simulink model "VehicleModel"  (R2016b)
settings: Solver=FixedStepAuto  StartTime=0.0  StopTime=t_EndSimulation  FixedStep=base_dT  MaxStep=0.01  RelTol=1e-3  EnableMultiTasking=on
values from neighbouring files (symbols this model uses):
  b_E2C_inloop = Simulink.Parameter    [VehicleModelInit.m]
  b_Engine_in_loop = Simulink.Parameter    [VehicleModelInit.m]
  b_initialize_distance_t_startsim = Simulink.Parameter    [VehicleModelInit.m]
  b_Ne_in_loop = Simulink.Parameter    [VehicleModelInit.m]
  b_TTB_in_loop = Simulink.Parameter    [VehicleModelInit.m]
  b_use_acc = Simulink.Parameter    [VehicleModelInit.m]
  b_use_acc_hardset = Simulink.Parameter    [VehicleModelInit.m]
  base_dT = Simulink.Parameter    [VehicleModelInit.m]
  c_acc_d_hdw = Simulink.Parameter    [VehicleModelInit.m]
  c_acc_hdw = Simulink.Parameter    [VehicleModelInit.m]
  c_EngFricCoef = PARS.c_EngFricCoef    [VehicleModelInit.m]
  c_EngFricCoefd = PARS.c_EngFricCoefd    [VehicleModelInit.m]
  d_Ne_max = Simulink.Parameter    [VehicleModelInit.m]
  d_Ne_min = Simulink.Parameter    [VehicleModelInit.m]
  Driver_TuneG1 = PARS.Driver_TuneG1    [VehicleModelInit.m]
  Driver_TuneG2 = PARS.Driver_TuneG2    [VehicleModelInit.m]
  Driver_TuneG3 = PARS.Driver_TuneG3    [VehicleModelInit.m]
  Driver_TuneG_aw = PARS.Driver_TuneG_aw    [VehicleModelInit.m]
  E2C_c2_dTB = Simulink.Parameter    [VehicleModelInit.m]
  E2C_c_dTB = Simulink.Parameter    [VehicleModelInit.m]
  E2C_CycleTimespan = Simulink.Parameter    [VehicleModelInit.m]
  E2C_initializeRelDist = Simulink.Parameter    [VehicleModelInit.m]
  E2C_SpeedShape = Simulink.Parameter    [VehicleModelInit.m]
  E2C_Trap_CycleAcceEndAlpha = Simulink.Parameter    [VehicleModelInit.m]
  E2C_Trap_CycleAcceStartAlpha = Simulink.Parameter    [VehicleModelInit.m]
  E2C_Trap_CycleDeceEndAlpha = Simulink.Parameter    [VehicleModelInit.m]
  E2C_Trap_CycleDeceStartAlpha = Simulink.Parameter    [VehicleModelInit.m]
  E2C_V_High_kmh = Simulink.Parameter    [VehicleModelInit.m]
  E2C_V_Low_kmh = Simulink.Parameter    [VehicleModelInit.m]
  E2C_V_max = Simulink.Parameter    [VehicleModelInit.m]
  E2C_V_min = Simulink.Parameter    [VehicleModelInit.m]
  FTP_speed_1sec = [FTP_speed_once.speed;Idle_speed_once;FTP_speed_once.speed;Idle_speed_once;FTP_speed_once.speed]    [VehicleModelInit.m]
  mass = 3123*1.3    (= 4059.9)    [VehicleModelInit.m]
  T_ACC_TuneG1_data = Simulink.Parameter    [VehicleModelInit.m]
  T_ACC_TuneG1_pt = Simulink.Parameter    [VehicleModelInit.m]
  T_ACC_TuneG2_data = Simulink.Parameter    [VehicleModelInit.m]
  T_ACC_TuneG2_pt = Simulink.Parameter    [VehicleModelInit.m]
  t_StartSimulation = Simulink.Parameter    [VehicleModelInit.m]
  T_TB_ego_ini = Simulink.Parameter    [VehicleModelInit.m]
  T_TB_OffSet = Simulink.Parameter    [VehicleModelInit.m]
  tau_EngTorque = Simulink.Parameter    [VehicleModelInit.m]
  tau_Ne = Simulink.Parameter    [VehicleModelInit.m]
  tau_pedal_dem = Simulink.Parameter    [VehicleModelInit.m]
  VESP_MD = x0.VESP    [VehicleModelInit.m]
undefined symbols (not defined in the file or in its folder): Continuous, DiscIntNeverNeededParam, initializeRelDist, p_ego_ini, p_lead_ini, PedalMapMD, r_w, Simulation_dT, spsSampleAndHoldModel, v_lead_ini, x0
libraries: simulink x9, spsEdgeDetectorModel x6, dspsigops x1
(part 2 of 7)

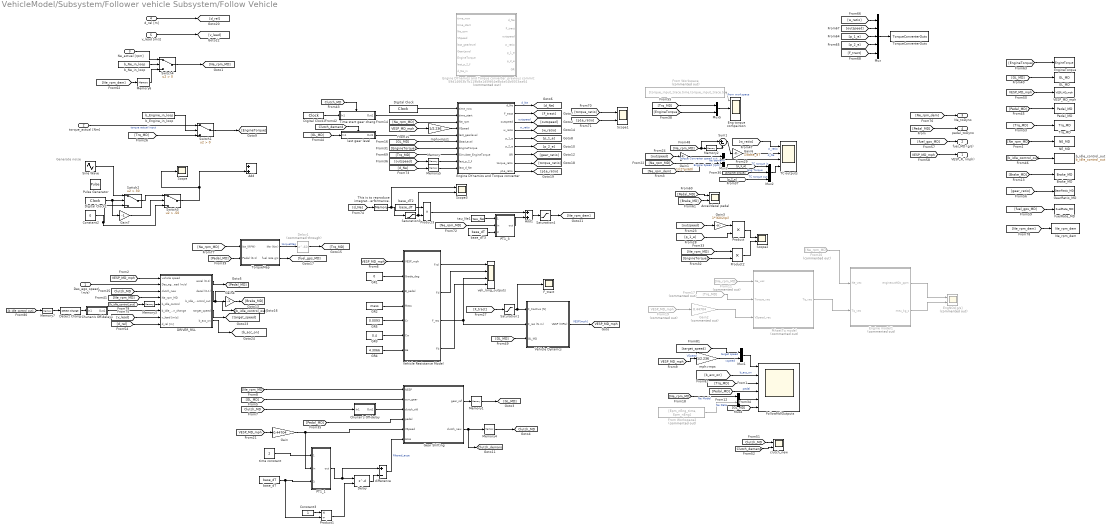
== system VehicleModel/Subsystem/Follower vehicle Subsystem/Follow Vehicle ==
  note: Generate noise
  Des_ego_speed (m/s) : Inport
  torque_actual [Nm] : Inport  Port=2
  Ne_actual [rpm] : Inport  Port=3
  d_rel [m] : Inport  Port=4
  v_lead [m/s] : Inport  Port=5
  Accel/decel pedal : Scope  NumInputPorts=2
  Add : Sum
  Add1 : Sum
  Brake_MD : ToWorkspace  VariableName=Brake_MD  SaveFormat=Structure With Time  SampleTime=-1
  Chunan's Off-delay : Subsystem
  Chunan's Off-delay1 : Subsystem
  Constant2 : Constant  Value=0
  Constant3 : Constant
  DRIVER_RSL : Subsystem
  Delay : Delay  DelayLengthSource=Input port  DelayLength=1
      settings: InputPortMap=u0,p1
  Delay1 : Delay  Commented=through  DelayLength=60
  Detect Change : simulink/Logic and Bit Operations/Detect Change  vinit=0  OutDataTypeStr=boolean
  Digital Clock : DigitalClock  SampleTime=-1
  Digital Clock1 : DigitalClock  SampleTime=-1
  Digital Clock2 : DigitalClock  SampleTime=-1
  Eng torque compairson : Scope  NumInputPorts=3
  EngNOx[g/s] : Scope  Commented=on  NumInputPorts=2
  Engine DYnamics and Torque converter : MATLAB Function  TreatAsAtomicUnit=on
  Engine DYnamics and Torque converter_previous commit: 59d14663b7b119b8a1d5fd64e8bda04b6003aa64 : MATLAB Function  Commented=on  TreatAsAtomicUnit=on
  Engine model1 : MATLAB Function  Commented=on  TreatAsAtomicUnit=on
  EngineTorque : ToWorkspace  VariableName=EngineTorque  SaveFormat=Structure With Time  SampleTime=-1
  F_tract : Scope
  FollowMdlOutputs : Scope  NumInputPorts=6
  From Workspace2 : FromWorkspace  Commented=on  VariableName=[Epm_nEng_time, Epm_nEng]
  From Workspace : FromWorkspace  Commented=on  VariableName=[torque_input_trace.time,torque_input_trace.tq]
  From11 : From  Commented=on  GotoTag=Ne_rpm_MD  TagVisibility=global
  From17 : From  Commented=on  GotoTag=Trq_MD  TagVisibility=global
  From19 : From  Commented=on  GotoTag=VESP_MD_mph  TagVisibility=global
  From20 : From  Commented=on  GotoTag=Ne_rpm_MD  TagVisibility=global
  FuelRate_MD : ToWorkspace  VariableName=FuelRate_MD  SaveFormat=Structure With Time  SampleTime=-1
  GL_MD : ToWorkspace  VariableName=GL_MD  SaveFormat=Structure With Time  SampleTime=-1
  GR1 : Constant  Value=0
  GR2 : Constant  Value=mass
  GR3 : Constant  Value=0.4
  GR4 : Constant  Value=4.3066
  GR5 : Constant  Value=0.0093
  Gain : Gain  Gain=0.44704
  Gain1 : Gain  Gain=1/(2*pi/60)
  Gain2 : Gain  Commented=on  Gain=0.44704
  Gain3 : Gain  Gain=1*(60/2/pi)
  Gain4 : Gain  Gain=-1
  Gain6 : Gain  Gain=1/base_dT
  Gain7 : Gain  Gain=-1
  Gear Shifting : MATLAB Function  TreatAsAtomicUnit=on
  GearRatio_MD : ToWorkspace  VariableName=GearRatio_MD  SaveFormat=Structure With Time  SampleTime=-1
  Memory{,3,5,7} (4 alike) : Memory  InheritSampleTime=on  LinearizeAsDelay=on
  Memory1 : Memory  X0=x0.GL  InheritSampleTime=on
  Memory2 : Memory  X0=600  InheritSampleTime=on  LinearizeAsDelay=on
  Memory4 : Memory  InheritSampleTime=on
  Memory6 : Memory  X0=600  InheritSampleTime=on  LinearizeAsDelay=on
  Mux : Mux  Inputs=5
  Mux1 : Mux  Inputs=2
  Mux2 : Mux  Inputs=3
  Mux3 : Mux  Inputs=3
  Mux4 : Mux  Inputs=2
  Mux5 : Mux  Inputs=2
  NE_MD : ToWorkspace  VariableName=NE_MD  SaveFormat=Structure With Time  SampleTime=-1
  Ne_rpm_dem : ToWorkspace  VariableName=Ne_rpm_dem  SaveFormat=Structure With Time  SampleTime=-1
  PT1_1 : Subsystem  mask(PT1_1){}
  PT1_3 : Subsystem  mask(PT1_1){}
  Pedal_MD : ToWorkspace  VariableName=Pedal_MD  SaveFormat=Structure With Time  SampleTime=-1
  Product : Product
  Product1 : Product  Inputs=*/
  Product2 : Product
  Product3 : Product
  PthsetTq model : MATLAB Function  Commented=on  TreatAsAtomicUnit=on
  Pulse Generator : DiscretePulseGenerator  Amplitude=250  Period=10  PulseWidth=5  SampleTime=-1
  Saturation1 : Saturate  UpperLimit=80000  LowerLimit=-80000
  Saturation3 : Saturate  UpperLimit=d_Ne_max  LowerLimit=d_Ne_min
  Saturation4 : Saturate  UpperLimit=3400  LowerLimit=600
  Scope : Scope
  Scope1 : Scope  NumInputPorts=2
  Scope2 : Scope  NumInputPorts=2
  Scope3 : Scope  NumInputPorts=2
  Sine Wave : Sin  Amplitude=0  Frequency=2
  Sum1 : Sum  Inputs=|+-
  Switch1 : Switch  Criteria=u2 > Threshold
  Switch2 : Switch  Criteria=u2 > Threshold  Threshold=30
  Switch3 : Switch  Criteria=u2 > Threshold  Threshold=-50
  Switch4 : Switch  Criteria=u2 > Threshold
  TC outputs : Scope  NumInputPorts=4
  This is to reproduce integrator performance. : Memory  InheritSampleTime=on  LinearizeAsDelay=on
  Time start gear change : Subsystem  TreatAsAtomicUnit=on
  TorqueConverterOuts : ToWorkspace  VariableName=TorqueConverterOuts  SaveFormat=Structure With Time  SampleTime=-1
  TorqueMap : Subsystem
  Trq_MD : ToWorkspace  VariableName=Trq_MD  SaveFormat=Structure With Time  SampleTime=-1
  VESP_MD_mph : ToWorkspace  VariableName=VESP_MD_mph  SaveFormat=Structure With Time  SampleTime=-1
  Vehicle Dynamcs : Subsystem
  Vehicle Resistance Model : MATLAB Function  TreatAsAtomicUnit=on
  b_Engine_in_loop : Constant  Value=b_Engine_in_loop
  b_Ne_in_loop : Constant  Value=b_Ne_in_loop
  b_idle_control_out : ToWorkspace  VariableName=b_idle_control_out  SaveFormat=Structure With Time  SampleTime=-1
  base_dT : Constant  Value=base_dT
  base_dT2 : Constant  Value=base_dT
  base_dT3 : Constant  Value=base_dT
  clutch_new : Scope  NumInputPorts=2
  difference : Sum  Inputs=+-  SaturateOnIntegerOverflow=on  InputSameDT=on  OutDataTypeStr=Inherit: Same as first input
  last gear level : Subsystem  TreatAsAtomicUnit=on
  mph>mps : Gain  Gain=1/2.236
  mph>mps1 : Gain  Gain=1/2.236
  tau_Ne1 : Constant  Value=tau_Ne
  time constant : Constant  Value=2
  veh_long_outputs : Scope  NumInputPorts=4
  VESP_FL (mph) : Outport
  fuel_MD (g/s) : Outport  Port=2
  Ne_toDyno : Outport  Port=3
  pedal_toDyno : Outport  Port=4
  tag scope: Clutch_MD=global, Clutch_demand=global, VESP_MD_mph=global
  wires:
  DRIVER_RSL/2(decel (0-1)) -> Gain4/1, Vehicle Resistance Model/3(B_pedal)
  Des_ego_speed (m/s)/1 -> DRIVER_RSL/2(Des_ego_speed (m/s))
  Vehicle Resistance Model/3(F_res) -> Vehicle Dynamcs/2(F_res (N.m)), veh_long_outputs/3
  GR1/1 -> Vehicle Resistance Model/2(Grade_deg)
  [VESP_MD_mph] -> Vehicle Resistance Model/1(VESP_mph)
  Vehicle Dynamcs/1(VESP (MPH)) -> [VESP_MD_mph]  "VESP[mph]"
  GR4/1 -> Vehicle Resistance Model/7(Aa)
  GR3/1 -> Vehicle Resistance Model/6(Cw)
  GR5/1 -> Vehicle Resistance Model/5(Cr)
  Vehicle Resistance Model/1(Frol) -> veh_long_outputs/1
  Vehicle Resistance Model/2(Fd) -> veh_long_outputs/2
  Vehicle Resistance Model/4(Fb) -> veh_long_outputs/4
  DRIVER_RSL/1(accel (0-1)) -> [Pedal_MD]
  [VESP_MD_mph] -> DRIVER_RSL/1(vehicle speed)
  [Ne_rpm_MD] -> TorqueMap/1(Ne_(RPM))
  TorqueMap/2(fuel rate g/s) -> [fuel_gps_MD]
  GR2/1 -> Vehicle Resistance Model/4(Mass)
  [GL_MD] -> Gear Shifting/2(curr_gear)
  [Ne_rpm_MD] -> Gear Shifting/1(NESP)
  Gear Shifting/1(gear_ref) -> Memory1/1
  Gear Shifting/2(clutch_new) -> Memory4/1, [Clutch_demand]
  [VESP_MD_mph] -> mph>mps/1  "VSpeed"
  [b_acc_on] -> FollowMdlOutputs/2  "b_acc_on"
  [Pedal_MD] -> FollowMdlOutputs/4  "pedal"
  Memory1/1 -> [GL_MD]
  [Trq_MD] -> FollowMdlOutputs/3
  Gain/1 -> PT1_1/2(in), Gear Shifting/5(VSpeed)
  [VESP_MD_mph] -> mph>mps1/1
  mph>mps1/1 -> Engine DYnamics and Torque converter/4(VSpeed)
  [GL_MD] -> Engine DYnamics and Torque converter/6(GearLevel)
  [EngineTorque] -> Mux2/2  "Eng Torque"
  Chunan's Off-delay/1(Out1) -> Gear Shifting/3(clutch_old)
  [Ne_rpm_MD] -> Engine DYnamics and Torque converter/3(Ne_rpm)
  [Ne_rpm_MD] -> Mux3/2  "Engine Speed [rpm]"
  Mux3/1 -> TC outputs/3
  From Workspace2/1 -> Mux4/2  "Ne Data"
  [Ne_rpm_MD] -> Mux4/1  "Ne Model"
  Mux4/1 -> FollowMdlOutputs/5
  From19/1 -> Gain2/1
  Gain2/1 -> PthsetTq model/3(VSpeed_vec)
  From17/1 -> PthsetTq model/2(Torque_vec)
  From11/1 -> PthsetTq model/1(Ne_vec)
  From20/1 -> Engine model1/1(Ne_vec)
  PthsetTq model/1(Tq_vec) -> Engine model1/2(Tq_vec)
  Engine model1/1(engineoutNOx_ppm) -> EngNOx[g/s]/1
  Engine model1/2(meu_kg_s) -> EngNOx[g/s]/2
  Engine DYnamics and Torque converter/1(d_Ne) -> [d_Ne]  "d_Ne"
  Engine DYnamics and Torque converter/3(outspeed) -> [outspeed]  "outspeed"
  [F_tract] -> Saturation1/1
  [VESP_MD_mph] -> Gain/1
  PT1_1/1(out) -> difference/1, Delay/1
  difference/1 -> Gear Shifting/6(Acce)  "filtered_acce"
  time constant/1 -> PT1_1/1(T_constant)
  Delay/1 -> difference/2
  Product1/1 -> Delay/2
  base_dT/1 -> Product1/2, PT1_1/3(T_sample)
  Constant3/1 -> Product1/1
  [Pedal_MD] -> pedal_toDyno/1
  Saturation1/1 -> F_tract/1, Vehicle Dynamcs/1(F_tractive [N])
  Product/1 -> Scope2/1
  Product2/1 -> Scope2/2
  Gain3/1 -> Product/1
  TorqueMap/1(Me (Nm)) -> Delay1/1  "torqueMap"
  b_Engine_in_loop/1 -> Switch1/2
  torque_actual [Nm]/1 -> Switch1/1  "torque actual input"
  [outspeed] -> Gain3/1
  [outspeed] -> Gain1/1
  Sum1/1 -> Gain6/1
  Engine DYnamics and Torque converter/2(F_tract) -> [F_tract]
  [p_1_e] -> Product/2
  [EngineTorque] -> Product2/2
  [Ne_rpm_MD] -> Product2/1
  [GL_MD] -> FollowMdlOutputs/6
  Gain4/1 -> [Brake_MD]
  [EngineTorque] -> Engine DYnamics and Torque converter/7(EngineTorque)
  Mux2/1 -> TC outputs/4
  [p_1_e] -> Mux2/1  "TC torque in"
  [p_2_e] -> Mux2/3  "TC torque out"
  Mux5/1 -> Eng torque compairson/2
  [Pedal_MD] -> TorqueMap/2(Pedal (0-1))
  [EngineTorque] -> Mux5/2
  From Workspace/1 -> Eng torque compairson/1  "from workspace"
  Gain1/1 -> Mux3/1  "Torque Converter speed out"
  [Ne_rpm_MD] -> Sum1/1, Memory2/1
  Memory2/1 -> Sum1/2
  [Clutch_MD] -> DRIVER_RSL/3(clutch_new)
  [Ne_rpm_MD] -> DRIVER_RSL/4(Ne_rpm_MD)
  Digital Clock/1 -> Engine DYnamics and Torque converter/1(time_now)
  [Clutch_MD] -> Chunan's Off-delay/1(In1)
  Memory4/1 -> [Clutch_MD]
  Digital Clock1/1 -> Time start gear change/1(In1)
  [Clutch_MD] -> Time start gear change/Trigger
  Time start gear change/1(Out1) -> Engine DYnamics and Torque converter/2(time_start)
  [Clutch_demand] -> last gear level/Trigger
  last gear level/1(Out1) -> Engine DYnamics and Torque converter/5(last_gearlevel)
  [GL_MD] -> last gear level/1(In1)
  [Trq_MD] -> Mux5/1
  Engine DYnamics and Torque converter/4(w_ratio) -> [w_ratio]  "w_ratio"
  [w_ratio] -> TC outputs/1  "w_ratio"
  Gain6/1 -> TC outputs/2  "d_Ne"
  [GL_MD] -> GL_MD/1
  [GL_MD] -> Vehicle Dynamcs/3(GL_MD)
  [VESP_MD_mph] -> VESP_MD_mph/1
  [Clutch_demand] -> clutch_new/2
  [Clutch_MD] -> clutch_new/1
  [Trq_MD] -> Trq_MD/1
  [Pedal_MD] -> Pedal_MD/1
  [Ne_rpm_MD] -> NE_MD/1
  [Brake_MD] -> Brake_MD/1
  [Pedal_MD] -> Gear Shifting/4(pedal)
  DRIVER_RSL/3(b_idle_control_out) -> [b_idle_control_out]
  [b_idle_control_out] -> b_idle_control_out/1
  [gear_ratio] -> GearRatio_MD/1
  [fuel_gps_MD] -> fuel_MD (g/s)/1
  [VESP_MD_mph] -> VESP_FL (mph)/1
  [fuel_gps_MD] -> FuelRate_MD/1
  [Brake_MD] -> Accel/decel pedal/2
  [Pedal_MD] -> Accel/decel pedal/1
  [Ne_rpm_dem] -> Ne_toDyno/1
  [Trq_MD] -> Switch1/3
  [EngineTorque] -> EngineTorque/1
  Mux/1 -> TorqueConverterOuts/1
  [w_ratio] -> Mux/1
  [outspeed] -> Mux/2
  [p_1_e] -> Mux/3
  [p_2_e] -> Mux/4
  [F_tract] -> Mux/5
  Digital Clock2/1 -> Gain7/1, Switch2/2
  Gain7/1 -> Switch3/2
  Sine Wave/1 -> Switch2/1
  Switch2/1 -> Switch3/1
  Constant2/1 -> Switch3/3, Switch2/3
  Switch3/1 -> Scope/1, Add/2
  Engine DYnamics and Torque converter/7(GR) -> [gear_ratio]
  Engine DYnamics and Torque converter/6(p_2_e) -> [p_2_e]
  Engine DYnamics and Torque converter/5(p_1_e) -> [p_1_e]
  Engine DYnamics and Torque converter/8(torque_ratio) -> [torque_ratio]
  Engine DYnamics and Torque converter/9(p1e_ratio) -> [p1e_ratio]
  [torque_ratio] -> Scope1/1
  [p1e_ratio] -> Scope1/2
  [outspeed] -> Memory/1
  Memory/1 -> Engine DYnamics and Torque converter/9(last_p_2_f)
  [d_Ne] -> Memory5/1
  Memory5/1 -> Engine DYnamics and Torque converter/10(last_d_Ne)
  [Trq_MD] -> Engine DYnamics and Torque converter/8(Simulate_EngineTorque)
  Switch1/1 -> [EngineTorque]
  [d_Ne] -> This is to reproduce integrator performance./1
  Product3/1 -> Add1/1
  Saturation3/1 -> Scope3/2, Product3/2
  base_dT2/1 -> Product3/1
  Add1/1 -> Saturation4/1
  Saturation4/1 -> [Ne_rpm_dem]
  [Ne_rpm_dem] -> Memory6/1
  This is to reproduce integrator performance./1 -> Scope3/1, Saturation3/1
  [Ne_rpm_dem] -> Mux3/3  "Ne demand"
  b_Ne_in_loop/1 -> Switch4/2
  Ne_actual [rpm]/1 -> Switch4/1
  Switch4/1 -> [Ne_rpm_MD]
  Memory6/1 -> Switch4/3
  [Ne_rpm_dem] -> Ne_rpm_dem/1
  tau_Ne1/1 -> PT1_3/1(T_constant)
  base_dT3/1 -> PT1_3/3(T_sample)
  [Ne_rpm_MD] -> PT1_3/2(in)
  PT1_3/1(out) -> Add1/2
  d_rel [m]/1 -> [d_rel]
  v_lead [m/s]/1 -> [v_lead]
  [d_rel] -> DRIVER_RSL/8(d_rel [m])
  [v_lead] -> DRIVER_RSL/7(v_lead [m/s])
  Chunan's Off-delay1/1(Out1) -> DRIVER_RSL/6(b_idle_is_in_change)
  Detect Change/1 -> Chunan's Off-delay1/1(In1)
  Delay1/1 -> [Trq_MD]
  [b_idle_control_out] -> Memory3/1
  Memory3/1 -> DRIVER_RSL/5(b_idle_control)
  [b_idle_control_out] -> Memory7/1
  Memory7/1 -> Detect Change/1
  DRIVER_RSL/4(target_speed) -> [target_speed]
  [target_speed] -> Mux1/1  "target speed"
  Mux1/1 -> FollowMdlOutputs/1
  mph>mps/1 -> Mux1/2  "vspeed"
  DRIVER_RSL/5("b_acc_on ") -> [b_acc_on]

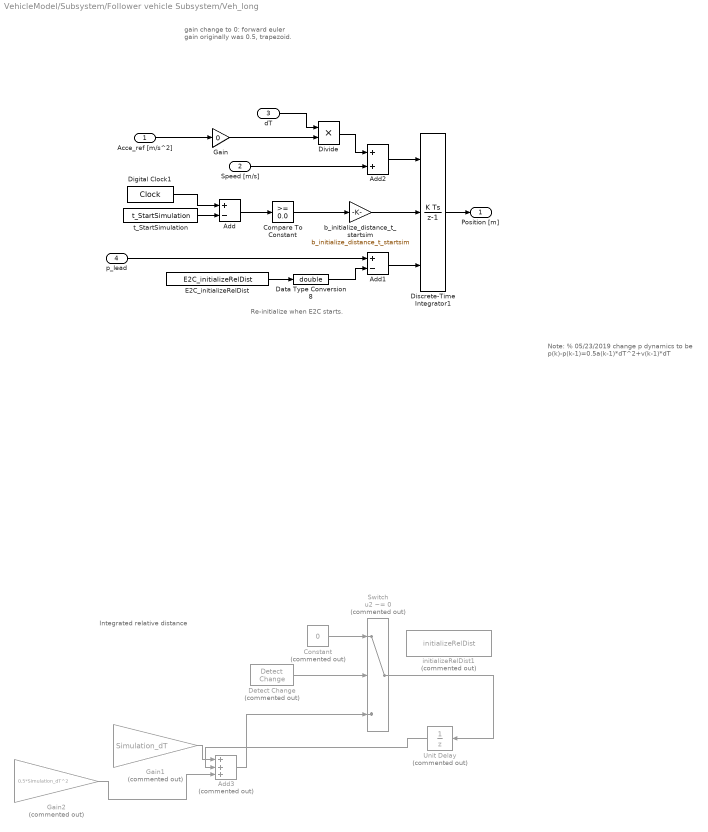
== system VehicleModel/Subsystem/Follower vehicle Subsystem/Veh_long  ==
  note: Re-initialize when E2C starts.
  note: gain change to 0: forward euler
      | gain originally was 0.5, trapezoid.
  note: Note:
      | % 05/23/2019
      | change p dynamics to be p(k)-p(k-1)=0.5a(k-1)*dT^2+v(k-1)*dT
  note: Integrated relative distance
  Acce_ref [m/s^2] : Inport
  Speed [m/s] : Inport  Port=2
  dT : Inport  Port=3
  p_lead : Inport  Port=4
  Add : Sum  Inputs=+-
  Add1 : Sum  Inputs=+-
  Add2 : Sum
  Add3 : Sum  Commented=on  Inputs=+++
  Compare To Constant : simulink/Logic and Bit Operations/Compare To Constant  relop=>=  const=0.0  OutDataTypeStr=uint8
  Constant : Constant  Commented=on  Value=0
  Data Type Conversion8 : DataTypeConversion  OutDataTypeStr=double
  Detect Change : simulink/Logic and Bit Operations/Detect Change  Commented=on  vinit=0  OutDataTypeStr=boolean
  Digital Clock1 : DigitalClock  SampleTime=-1
  Discrete-Time Integrator1 : DiscreteIntegrator  ExternalReset=rising  InitialConditionSource=external  InitialCondition=p_ego_ini  SampleTime=-1  ICPrevOutput=DiscIntNeverNeededParam  ICPrevScaledInput=DiscIntNeverNeededParam
  Divide : Product  Inputs=**
  E2C_initializeRelDist : Constant  Value=E2C_initializeRelDist  OutDataTypeStr=double
  Gain : Gain  Gain=0
  Gain1 : Gain  Commented=on  Gain=Simulation_dT
  Gain2 : Gain  Commented=on  Gain=0.5*Simulation_dT^2
  Switch : Switch  Commented=on  Criteria=u2 ~= 0
  Unit Delay : UnitDelay  Commented=on  SampleTime=-1
  b_initialize_distance_t_startsim : Gain  Gain=b_initialize_distance_t_startsim
  initializeRelDist1 : Constant  Commented=on  Value=initializeRelDist
  t_StartSimulation : Constant  Value=t_StartSimulation
  Position [m] : Outport
  wires:
  Divide/1 -> Add2/1
  Add2/1 -> Discrete-Time Integrator1/1
  Switch/1 -> Unit Delay/1
  Detect Change/1 -> Switch/2
  Add3/1 -> Switch/3
  Unit Delay/1 -> Add3/2
  Gain1/1 -> Add3/1
  Constant/1 -> Switch/1
  Gain2/1 -> Add3/3
  Discrete-Time Integrator1/1 -> Position [m]/1
  Add1/1 -> Discrete-Time Integrator1/3
  Speed [m/s]/1 -> Add2/2
  Acce_ref [m/s^2]/1 -> Gain/1
  E2C_initializeRelDist/1 -> Data Type Conversion8/1
  Gain/1 -> Divide/2
  dT/1 -> Divide/1
  Add/1 -> Compare To Constant/1
  t_StartSimulation/1 -> Add/2
  Digital Clock1/1 -> Add/1
  Compare To Constant/1 -> b_initialize_distance_t_startsim/1
  p_lead/1 -> Add1/1
  Data Type Conversion8/1 -> Add1/2
  b_initialize_distance_t_startsim/1 -> Discrete-Time Integrator1/2

== system VehicleModel/Subsystem/Lead_Veh_long/noequal ==
  In1 : Inport
  Relational Operator : RelationalOperator  Operator=~=  OutDataTypeStr=boolean  RndMeth=Simplest
  Unit Delay : UnitDelay  SampleTime=-1
  Out1 : Outport
  wires:
  Relational Operator/1 -> Out1/1
  Unit Delay/1 -> Relational Operator/2
  In1/1 -> Unit Delay/1, Relational Operator/1

== system VehicleModel/Subsystem/Follower vehicle Subsystem/Follow Vehicle/Chunan's Off-delay ==
  In1 : Inport
  Constant : Constant
  Constant2 : Constant  Value=0
  Data Type Conversion1 : DataTypeConversion  OutDataTypeStr=boolean  SaturateOnIntegerOverflow=on  RndMeth=Zero
  Digital Clock : DigitalClock  SampleTime=-1
  Logical Operator4 : Logic  Operator=NOT  Inputs=1
  OFF Delay : Subsystem  AncestorBlock=spsOnOffDelayModel/Continuous/OFF Delay  TreatAsAtomicUnit=on
  Relational Operator1 : RelationalOperator  Operator===  RndMeth=Nearest  InputSameDT=on
  delay length : Constant  Value=2
  Out1 : Outport
  wires:
  OFF Delay/1(OUT) -> Out1/1
  Logical Operator4/1 -> OFF Delay/Enable
  Constant2/1 -> Relational Operator1/1
  Relational Operator1/1 -> Logical Operator4/1
  Constant/1 -> Relational Operator1/2
  Data Type Conversion1/1 -> OFF Delay/1(IN)
  Digital Clock/1 -> OFF Delay/2(clock)
  delay length/1 -> OFF Delay/3(DELAY)
  In1/1 -> Data Type Conversion1/1

== system VehicleModel/Subsystem/Follower vehicle Subsystem/Follow Vehicle/Chunan's Off-delay1 ==
  In1 : Inport
  Constant : Constant
  Constant2 : Constant  Value=0
  Data Type Conversion1 : DataTypeConversion  OutDataTypeStr=boolean  SaturateOnIntegerOverflow=on  RndMeth=Zero
  Digital Clock : DigitalClock  SampleTime=-1
  Logical Operator4 : Logic  Operator=NOT  Inputs=1
  OFF Delay : Subsystem  AncestorBlock=spsOnOffDelayModel/Continuous/OFF Delay  TreatAsAtomicUnit=on
  Relational Operator1 : RelationalOperator  Operator===  RndMeth=Nearest  InputSameDT=on
  delay length : Constant
  Out1 : Outport
  wires:
  OFF Delay/1(OUT) -> Out1/1
  Logical Operator4/1 -> OFF Delay/Enable
  Constant2/1 -> Relational Operator1/1
  Relational Operator1/1 -> Logical Operator4/1
  Constant/1 -> Relational Operator1/2
  Data Type Conversion1/1 -> OFF Delay/1(IN)
  Digital Clock/1 -> OFF Delay/2(clock)
  delay length/1 -> OFF Delay/3(DELAY)
  In1/1 -> Data Type Conversion1/1

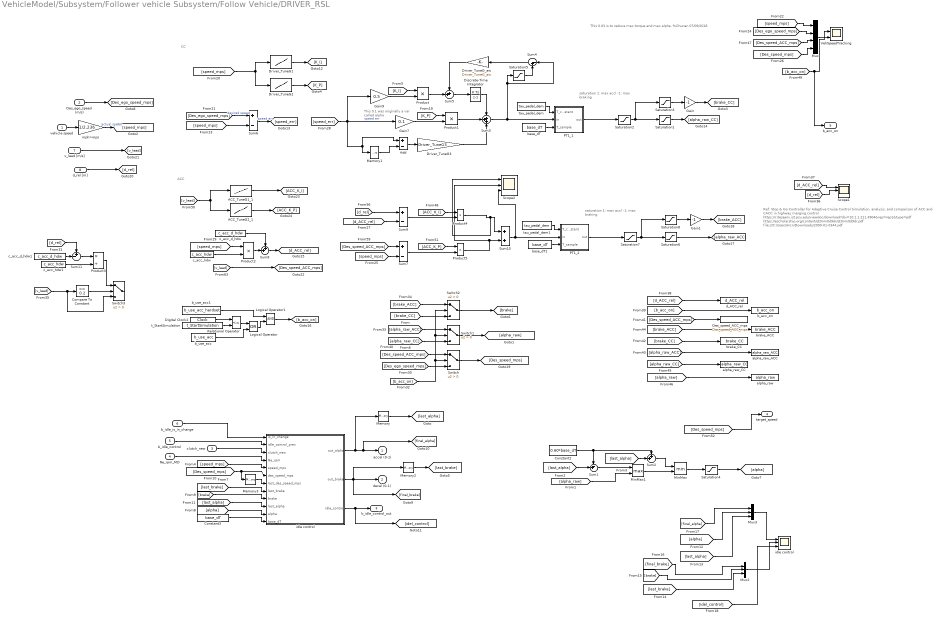
== system VehicleModel/Subsystem/Follower vehicle Subsystem/Follow Vehicle/DRIVER_RSL ==
  note: ACC
  note: CC
  note: Ref:
      | Stop & Go Controller for Adaptive Cruise Control
      | Simulation, analysis, and comparison of ACC and CACC in highway merging control
      | https://citeseerx.ist.psu.edu/viewdoc/download?doi=10.1.1.211.4904&rep=rep1&type=pdf
      | https://escholarship.org/content/qt0nm0d9dr/qt0nm0d9dr.pdf
      | file:///C:/Users/Hcn/Downloads/2000-01-0344.pdf
  note: This 0.1 was originally a var called alpha
  note: saturation
      | 1: max accl
      | -1: max braking
  note: This 0.03 is to reduce max torque and max alpha. %Chunan 07/09/2018
  note: saturation
      | 1: max accl
      | -1: max braking
  vehicle speed : Inport
  Des_ego_speed (m/s) : Inport  Port=2
  clutch_new : Inport  Port=3
  Ne_rpm_MD : Inport  Port=4
  b_idle_control : Inport  Port=5
  b_idle_is_in_change : Inport  Port=6
  v_lead [m/s] : Inport  Port=7
  d_rel [m] : Inport  Port=8
  ACC_TuneG1_1 : Lookup_n-D  NumberOfTableDimensions=1  BreakpointsForDimension1=T_ACC_TuneG1_pt  Table=T_ACC_TuneG1_data  InternalRulePriority=Speed  RndMeth=Simplest  InputSameDT=on
  ACC_TuneG2_1 : Lookup_n-D  NumberOfTableDimensions=1  BreakpointsForDimension1=T_ACC_TuneG2_pt  Table=T_ACC_TuneG2_data  InternalRulePriority=Speed  RndMeth=Simplest  InputSameDT=on
  Add : Sum  Inputs=+-
  Compare To Constant : simulink/Logic and Bit Operations/Compare To Constant  relop=>=  const=0.2  OutDataTypeStr=boolean
  Constant2 : Constant  Value=0.60*base_dT
  Constant3 : Constant  Value=base_dT
  Des_speed_ACC_mps : ToWorkspace  VariableName=Des_speed_ACC_mps  SaveFormat=Structure With Time  SampleTime=-1
  Digital Clock2 : DigitalClock  SampleTime=-1
  Discrete-Time Integrator : DiscreteIntegrator  gainval=1  InitialConditionSetting=State (most efficient)  SampleTime=-1  ICPrevOutput=DiscIntNeverNeededParam  ICPrevScaledInput=DiscIntNeverNeededParam
  Driver_TuneG1 : Lookup_n-D  NumberOfTableDimensions=1  BreakpointsForDimension1=[-1, 0.5, 3, 8.1, 50]  Table=[Driver_TuneG1*3,Driver_TuneG1*2.5, Driver_TuneG1*2, Driver_TuneG1, Driver_TuneG1]  InternalRulePriority=Speed  RndMeth=Simplest  InputSameDT=on
  Driver_TuneG2 : Lookup_n-D  NumberOfTableDimensions=1  BreakpointsForDimension1=[-1,0.5, 3, 8.1, 50]  Table=[Driver_TuneG2*6, Driver_TuneG2*3, Driver_TuneG2*2, Driver_TuneG2, Driver_TuneG2]  InternalRulePriority=Speed  RndMeth=Simplest  InputSameDT=on
  Driver_TuneG3 : Gain  Gain=Driver_TuneG3  SaturateOnIntegerOverflow=on  OutDataTypeStr=Inherit: Same as input  ParamDataTypeStr=Inherit: Same as input
  Driver_TuneG_aw : Gain  Gain=Driver_TuneG_aw
  Gain : Gain  Gain=-1  SaturateOnIntegerOverflow=on  OutDataTypeStr=Inherit: Same as input  ParamDataTypeStr=Inherit: Same as input
  Gain1 : Gain  Gain=-1  SaturateOnIntegerOverflow=on  OutDataTypeStr=Inherit: Same as input  ParamDataTypeStr=Inherit: Same as input
  Gain7 : Gain  Gain=0.1  SaturateOnIntegerOverflow=on  OutDataTypeStr=Inherit: Same as input  ParamDataTypeStr=Inherit: Same as input
  Gain9 : Gain  Gain=0.5  SaturateOnIntegerOverflow=on  OutDataTypeStr=Inherit: Same as input  ParamDataTypeStr=Inherit: Same as input
  Logical Operator : Logic  Operator=OR  AllPortsSameDT=off  OutDataTypeStr=boolean
  Logical Operator1 : Logic  AllPortsSameDT=off  OutDataTypeStr=boolean
  Memory{,1..3} (4 alike) : Memory  InheritSampleTime=on  LinearizeAsDelay=on
  MinMax : MinMax  Inputs=2
  MinMax1 : MinMax  Function=max  Inputs=2
  Mux : Mux
  Mux2 : Mux  Inputs=3
  Mux3 : Mux  Inputs=3
  PT1_1 : Subsystem  mask(PT1_1){}
  PT1_2 : Subsystem  mask(PT1_1){}
  Product{,1,4..5} (4 alike) : Product
  Product2 : Product  Inputs=**
  Product3 : Product  Inputs=*/
  Relational Operator : RelationalOperator  Operator=<=  OutDataTypeStr=boolean  RndMeth=Simplest
  Saturation1 : Saturate  UpperLimit=1  LowerLimit=0
  Saturation2 : Saturate  UpperLimit=1  LowerLimit=-1
  Saturation3 : Saturate  UpperLimit=0  LowerLimit=-1
  Saturation4 : Saturate  UpperLimit=1  LowerLimit=0
  Saturation5 : Saturate  UpperLimit=1  LowerLimit=-1
  Saturation6 : Saturate  UpperLimit=1  LowerLimit=0
  Saturation7 : Saturate  UpperLimit=1  LowerLimit=-1
  Saturation8 : Saturate  UpperLimit=0  LowerLimit=-1
  Scope1 : Scope  NumInputPorts=3
  Scope2 : Scope  NumInputPorts=3
  Sum1 : Sum  Inputs=-+|
  Sum10 : Sum  SaturateOnIntegerOverflow=on  InputSameDT=on  OutDataTypeStr=Inherit: Same as first input
  Sum11 : Sum  Inputs=+-|
  Sum2 : Sum  Inputs=++|
  Sum3 : Sum  Inputs=+++
  Sum4 : Sum  Inputs=|-+
  Sum5 : Sum  Inputs=++|
  Sum6 : Sum  Inputs=+-  SaturateOnIntegerOverflow=on  InputSameDT=on  OutDataTypeStr=Inherit: Same as first input
  Sum7 : Sum  Inputs=+-  SaturateOnIntegerOverflow=on  InputSameDT=on  OutDataTypeStr=Inherit: Same as first input
  Sum8 : Sum  Inputs=++|
  Sum9 : Sum  Inputs=+-  SaturateOnIntegerOverflow=on  InputSameDT=on  OutDataTypeStr=Inherit: Same as first input
  Switch{,1..3} (4 alike) : Switch  Criteria=u2 > Threshold
  VehSpeedTracking : Scope  NumInputPorts=2
  alpha_raw : ToWorkspace  VariableName=alpha_raw  SaveFormat=Structure With Time  SampleTime=-1
  alpha_raw_ACC : ToWorkspace  VariableName=alpha_raw_ACC  SaveFormat=Structure With Time  SampleTime=-1
  alpha_raw_CC : ToWorkspace  VariableName=alpha_raw_CC  SaveFormat=Structure With Time  SampleTime=-1
  b_acc_on : ToWorkspace  VariableName=b_acc_on  SaveFormat=Structure With Time  SampleTime=-1
  b_use_acc : Constant  Value=b_use_acc
  b_use_acc1 : Constant  Value=b_use_acc_hardset
  base_dT : Constant  Value=base_dT
  base_dT1 : Constant  Value=base_dT
  brake_ACC : ToWorkspace  VariableName=brake_ACC  SaveFormat=Structure With Time  SampleTime=-1
  brake_CC : ToWorkspace  VariableName=brake_CC  SaveFormat=Structure With Time  SampleTime=-1
  c_acc_d_hdw : Constant  Value=c_acc_d_hdw
  c_acc_d_hdw1 : Constant  Value=c_acc_d_hdw
  c_acc_hdw : Constant  Value=c_acc_hdw
  c_acc_hdw1 : Constant  Value=c_acc_hdw
  d_ACC_rel : ToWorkspace  VariableName=d_ACC_rel  SaveFormat=Structure With Time  SampleTime=-1
  idle control : MATLAB Function  TreatAsAtomicUnit=on
  "idle control " : Scope  NumInputPorts=3
  mph>mps : Gain  Gain=1/2.236
  t_StartSimulation : Constant  Value=t_StartSimulation
  tau_pedal_dem : Constant  Value=tau_pedal_dem
  tau_pedal_dem1 : Constant  Value=tau_pedal_dem
  accel (0-1) : Outport
  decel (0-1) : Outport  Port=2
  b_idle_control_out : Outport  Port=3
  target_speed : Outport  Port=4
  "b_acc_on " : Outport  Port=5
  wires:
  Gain/1 -> [brake_CC]
  Saturation3/1 -> Gain/1
  Saturation1/1 -> [alpha_raw_CC]
  vehicle speed/1 -> mph>mps/1
  Mux/1 -> VehSpeedTracking/1
  Saturation2/1 -> Saturation3/1, Saturation1/1
  Gain7/1 -> Product1/2
  Gain9/1 -> Product/2
  [Des_ego_speed_mps] -> Sum6/1  "desired speed"
  mph>mps/1 -> [speed_mps]  "actual speed"
  [speed_err] -> Gain7/1, Add/1, Memory1/1, Gain9/1  "speed err"
  Product/1 -> Sum5/2
  tau_pedal_dem/1 -> PT1_1/1(T_constant)
  base_dT/1 -> PT1_1/3(T_sample)
  PT1_1/1(out) -> Saturation2/1
  Memory/1 -> [last_alpha]
  MinMax/1 -> Saturation4/1
  [alpha_raw] -> MinMax1/2
  Saturation4/1 -> [alpha]
  [last_alpha] -> Sum1/2
  Constant2/1 -> Sum1/1, Sum2/1
  Sum1/1 -> MinMax1/1
  [last_alpha] -> Sum2/2
  MinMax1/1 -> MinMax/2
  Sum2/1 -> MinMax/1
  Memory1/1 -> Add/2
  Add/1 -> Driver_TuneG3/1
  Driver_TuneG3/1 -> Sum3/3
  Product1/1 -> Sum3/2
  Discrete-Time Integrator/1 -> Sum3/1
  Sum3/1 -> Sum4/1, Saturation5/1, PT1_1/2(in)
  Saturation5/1 -> Sum4/2
  Sum4/1 -> Driver_TuneG_aw/1
  Driver_TuneG_aw/1 -> Sum5/1
  Sum5/1 -> Discrete-Time Integrator/1
  Memory2/1 -> [last_brake]
  [alpha] -> idle control/11(alpha)
  [last_brake] -> idle control/8(last_brake)
  [speed_mps] -> idle control/5(speed_mps)
  Ne_rpm_MD/1 -> idle control/4(Ne_rpm)
  clutch_new/1 -> idle control/3(clutch_new)
  b_idle_control/1 -> idle control/2(idle_control_prev)
  [brake] -> idle control/9(brake)
  [Des_speed_mps] -> Memory3/1, idle control/6(des_speed_mps)
  [last_alpha] -> idle control/10(last_alpha)
  Constant3/1 -> idle control/12(base_dT)
  idle control/1(out_alpha) -> Memory/1, [final_alpha], accel (0-1)/1
  idle control/2(out_brake) -> [final_brake], Memory2/1, decel (0-1)/1
  idle control/3(idle_control) -> [idel_control], b_idle_control_out/1
  Mux2/1 -> "idle control "/2
  [final_brake] -> Mux2/1
  [brake] -> Mux2/2
  [last_brake] -> Mux2/3
  Mux3/1 -> "idle control "/1
  [last_alpha] -> Mux3/3
  [alpha] -> Mux3/2
  [final_alpha] -> Mux3/1
  [idel_control] -> "idle control "/3
  Memory3/1 -> idle control/7(last_des_speed_mps)
  Driver_TuneG1/1 -> [K_I]
  [K_I] -> Product/1
  Driver_TuneG2/1 -> [K_P]
  [K_P] -> Product1/1
  [speed_mps] -> Driver_TuneG2/1, Driver_TuneG1/1
  Des_ego_speed (m/s)/1 -> [Des_ego_speed_mps]
  [speed_mps] -> Mux/1
  [speed_mps] -> Sum6/2
  [Des_ego_speed_mps] -> Mux/2
  Sum6/1 -> [speed_err]  "speed err"
  Switch2/1 -> [brake]
  Switch1/1 -> [alpha_raw]
  [speed_mps] -> Sum7/2
  c_acc_hdw/1 -> Product2/2
  Sum8/1 -> [d_ACC_rel]
  c_acc_d_hdw/1 -> Sum8/1
  [speed_mps] -> Product2/1
  Product2/1 -> Sum8/2
  t_StartSimulation/1 -> Relational Operator/2
  Digital Clock2/1 -> Relational Operator/1
  Relational Operator/1 -> Logical Operator/1
  b_use_acc/1 -> Logical Operator/2
  Logical Operator/1 -> Logical Operator1/2
  b_use_acc1/1 -> Logical Operator1/1
  [d_ACC_rel] -> Sum9/2
  Sum9/1 -> Product4/2
  Sum7/1 -> Product5/2
  Product4/1 -> Scope2/1, Sum10/1
  Product5/1 -> Sum10/2, Scope2/2
  Gain1/1 -> [brake_ACC]
  Saturation8/1 -> Gain1/1
  Saturation6/1 -> [alpha_raw_ACC]
  Saturation7/1 -> Saturation8/1, Saturation6/1
  tau_pedal_dem1/1 -> PT1_2/1(T_constant)
  base_dT1/1 -> PT1_2/3(T_sample)
  PT1_2/1(out) -> Saturation7/1
  Sum10/1 -> Scope2/3, PT1_2/2(in)
  Sum11/1 -> Product3/1
  c_acc_d_hdw1/1 -> Sum11/2
  [d_rel] -> Sum11/1
  c_acc_hdw1/1 -> Product3/2
  Switch/1 -> [Des_speed_mps]
  [Des_ego_speed_mps] -> Switch/3
  [v_lead] -> [Des_speed_ACC_mps]
  [b_acc_on] -> Switch1/2, Switch2/2, Switch/2
  [alpha_raw_CC] -> Switch1/3
  [alpha_raw_ACC] -> Switch1/1
  [brake_CC] -> Switch2/3
  [brake_ACC] -> Switch2/1
  Product3/1 -> Switch3/1
  [v_lead] -> Switch3/3, Compare To Constant/1
  Compare To Constant/1 -> Switch3/2
  [d_rel] -> Scope1/2
  [d_ACC_rel] -> Scope1/1
  b_idle_is_in_change/1 -> idle control/1(is_in_change)
  Logical Operator1/1 -> [b_acc_on]
  [Des_speed_ACC_mps] -> Switch/1
  [d_ACC_rel] -> d_ACC_rel/1
  [b_acc_on] -> b_acc_on/1
  [Des_speed_ACC_mps] -> Des_speed_ACC_mps/1
  [brake_ACC] -> brake_ACC/1
  [brake_CC] -> brake_CC/1
  [alpha_raw_ACC] -> alpha_raw_ACC/1
  [alpha_raw_CC] -> alpha_raw_CC/1
  [alpha_raw] -> alpha_raw/1
  [Des_speed_ACC_mps] -> Mux/3
  [Des_speed_mps] -> Mux/4
  [b_acc_on] -> "b_acc_on "/1, VehSpeedTracking/2
  [v_lead] -> ACC_TuneG1_1/1, ACC_TuneG2_1/1
  ACC_TuneG1_1/1 -> [ACC_K_I]
  [ACC_K_I] -> Product4/1
  ACC_TuneG2_1/1 -> [ACC_K_P]
  [ACC_K_P] -> Product5/1
  v_lead [m/s]/1 -> [v_lead]
  [Des_speed_ACC_mps] -> Sum7/1
  d_rel [m]/1 -> [d_rel]
  [d_rel] -> Sum9/1
  [Des_speed_mps] -> target_speed/1

== system VehicleModel/Subsystem/Follower vehicle Subsystem/Follow Vehicle/PT1_1 ==
  T_constant : Inport
  in : Inport  Port=2
  T_sample : Inport  Port=3
  map_error_1 : Sum  Inputs=+-  SaturateOnIntegerOverflow=on  InputSameDT=on  OutDataTypeStr=Inherit: Same as first input
  map_error_2 : Sum  Inputs=2  SaturateOnIntegerOverflow=on  InputSameDT=on  OutDataTypeStr=Inherit: Same as first input
  product_1 : Product  Inputs=*/  SaturateOnIntegerOverflow=on  InputSameDT=on  OutDataTypeStr=Inherit: Same as first input
  product_2 : Product  Inputs=**  SaturateOnIntegerOverflow=on  InputSameDT=on  OutDataTypeStr=Inherit: Same as first input
  saturation_1 : Saturate  UpperLimit=1  LowerLimit=0
  unit_delay_1 : UnitDelay  SampleTime=-1
  out : Outport
  wires:
  T_constant/1 -> product_1/2
  T_sample/1 -> product_1/1
  in/1 -> map_error_1/1
  map_error_1/1 -> product_2/2
  product_1/1 -> saturation_1/1
  saturation_1/1 -> product_2/1
  unit_delay_1/1 -> map_error_1/2, map_error_2/2
  map_error_2/1 -> out/1, unit_delay_1/1
  product_2/1 -> map_error_2/1

== system VehicleModel/Subsystem/Follower vehicle Subsystem/Follow Vehicle/PT1_3 ==
  T_constant : Inport
  in : Inport  Port=2
  T_sample : Inport  Port=3
  map_error_1 : Sum  Inputs=+-  SaturateOnIntegerOverflow=on  InputSameDT=on  OutDataTypeStr=Inherit: Same as first input
  map_error_2 : Sum  Inputs=2  SaturateOnIntegerOverflow=on  InputSameDT=on  OutDataTypeStr=Inherit: Same as first input
  product_1 : Product  Inputs=*/  SaturateOnIntegerOverflow=on  InputSameDT=on  OutDataTypeStr=Inherit: Same as first input
  product_2 : Product  Inputs=**  SaturateOnIntegerOverflow=on  InputSameDT=on  OutDataTypeStr=Inherit: Same as first input
  saturation_1 : Saturate  UpperLimit=1  LowerLimit=0
  unit_delay_1 : UnitDelay  SampleTime=-1
  out : Outport
  wires:
  T_constant/1 -> product_1/2
  T_sample/1 -> product_1/1
  in/1 -> map_error_1/1
  map_error_1/1 -> product_2/2
  product_1/1 -> saturation_1/1
  saturation_1/1 -> product_2/1
  unit_delay_1/1 -> map_error_1/2, map_error_2/2
  map_error_2/1 -> out/1, unit_delay_1/1
  product_2/1 -> map_error_2/1

== system VehicleModel/Subsystem/Follower vehicle Subsystem/Follow Vehicle/Time start gear change ==
  In1 : Inport
  Trigger : TriggerPort  VariantControl=Variant
  Out1 : Outport
  wires:
  In1/1 -> Out1/1

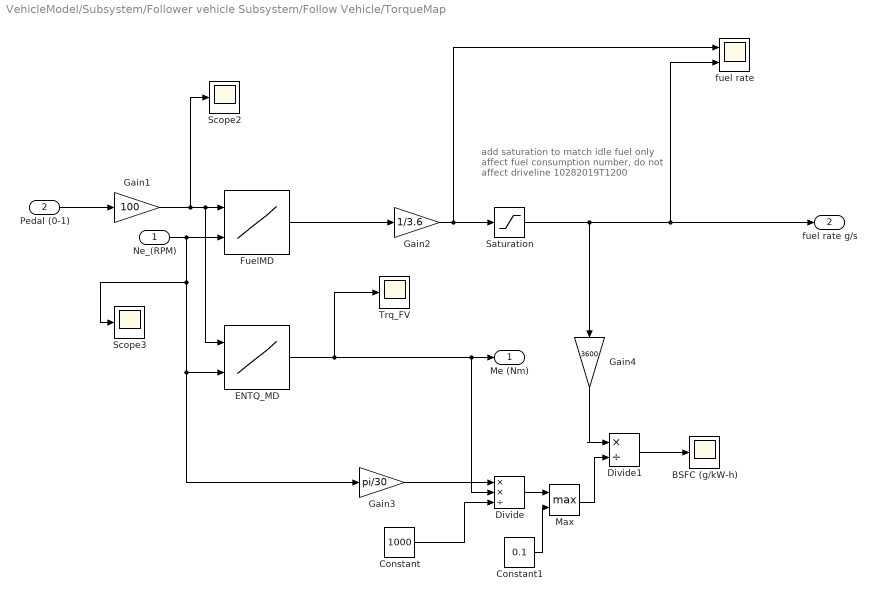
== system VehicleModel/Subsystem/Follower vehicle Subsystem/Follow Vehicle/TorqueMap ==
  note: add saturation to match idle fuel
      | only affect fuel consumption number,
      | do not affect driveline
      | 10282019T1200
  Ne_(RPM) : Inport
  Pedal (0-1) : Inport  Port=2
  BSFC (g/kW-h) : Scope
  Constant : Constant  Value=1000
  Constant1 : Constant  Value=0.1
  Divide : Product  Inputs=**/
  Divide1 : Product  Inputs=*/
  ENTQ_MD : Lookup_n-D  BreakpointsForDimension1=PedalMapMD.X  BreakpointsForDimension2=PedalMapMD.Y  Table=PedalMapMD.Torque'  ExtrapMethod=Clip  UseLastTableValue=on  InternalRulePriority=Speed  RndMeth=Simplest  InputSameDT=on
  FuelMD : Lookup_n-D  BreakpointsForDimension1=PedalMapMD.X  BreakpointsForDimension2=PedalMapMD.Y  Table=PedalMapMD.Fuel'  ExtrapMethod=Clip  UseLastTableValue=on  InternalRulePriority=Speed  RndMeth=Simplest  InputSameDT=on
  Gain1 : Gain  Gain=100  SaturateOnIntegerOverflow=on  OutDataTypeStr=Inherit: Same as input  ParamDataTypeStr=Inherit: Same as input
  Gain2 : Gain  Gain=1/3.6  SaturateOnIntegerOverflow=on  OutDataTypeStr=Inherit: Same as input  ParamDataTypeStr=Inherit: Same as input
  Gain3 : Gain  Gain=pi/30  SaturateOnIntegerOverflow=on  OutDataTypeStr=Inherit: Same as input  ParamDataTypeStr=Inherit: Same as input
  Gain4 : Gain  Gain=3600  SaturateOnIntegerOverflow=on  OutDataTypeStr=Inherit: Same as input  ParamDataTypeStr=Inherit: Same as input
  Max : MinMax  Function=max  Inputs=2
  Saturation : Saturate  UpperLimit=20  LowerLimit=0.2
  Scope2 : Scope
  Scope3 : Scope
  Trq_FV : Scope
  fuel rate : Scope  NumInputPorts=2
  Me (Nm) : Outport
  fuel rate g/s : Outport  Port=2
  wires:
  ENTQ_MD/1 -> Divide/2, Me (Nm)/1, Trq_FV/1
  Ne_(RPM)/1 -> Gain3/1, ENTQ_MD/2, Scope3/1, FuelMD/2
  Pedal (0-1)/1 -> Gain1/1
  Gain1/1 -> Scope2/1, ENTQ_MD/1, FuelMD/1
  FuelMD/1 -> Gain2/1
  Gain2/1 -> fuel rate/1, Saturation/1
  Gain3/1 -> Divide/1
  Constant/1 -> Divide/3
  Divide/1 -> Max/1
  Divide1/1 -> BSFC (g/kW-h)/1
  Gain4/1 -> Divide1/1
  Max/1 -> Divide1/2
  Constant1/1 -> Max/2
  Saturation/1 -> fuel rate/2, fuel rate g/s/1, Gain4/1

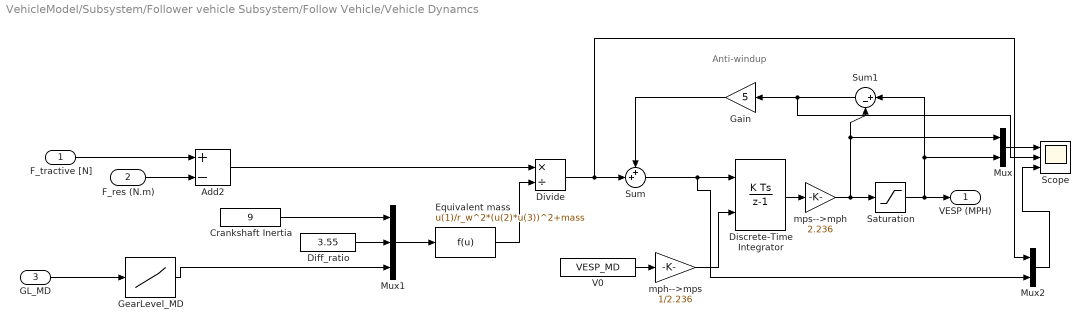
== system VehicleModel/Subsystem/Follower vehicle Subsystem/Follow Vehicle/Vehicle Dynamcs ==
  note: Anti-windup
  F_tractive [N] : Inport
  F_res (N.m) : Inport  Port=2
  GL_MD : Inport  Port=3
  Add2 : Sum  Inputs=+-
  Crankshaft Inertia : Constant  Value=9
  Diff_ratio : Constant  Value=3.55
  Discrete-Time Integrator : DiscreteIntegrator  InitialConditionSource=external  InitialConditionSetting=State (most efficient)  SampleTime=-1  ICPrevOutput=DiscIntNeverNeededParam  ICPrevScaledInput=DiscIntNeverNeededParam
  Divide : Product  Inputs=*/
  Equivalent mass : Fcn  Expr=u(1)/r_w^2*(u(2)*u(3))^2+mass
  Gain : Gain  Gain=5
  GearLevel_MD : Lookup_n-D  NumberOfTableDimensions=1  BreakpointsForDimension1=[1,2,3,4,5,6]  Table=[3.974,2.318,1.516,1.149,0.858,0.674]  ExtrapMethod=Clip  UseLastTableValue=on  InternalRulePriority=Speed  RndMeth=Simplest  InputSameDT=on
  Mux : Mux  Inputs=2
  Mux1 : Mux  Inputs=3
  Mux2 : Mux  Inputs=2
  Saturation : Saturate  UpperLimit=100  LowerLimit=0
  Scope : Scope  NumInputPorts=3
  Sum : Sum  Inputs=++|
  Sum1 : Sum  Inputs=|+-
  V0 : Constant  Value=VESP_MD
  mph-->mps : Gain  Gain=1/2.236
  mps-->mph : Gain  Gain=2.236
  VESP (MPH) : Outport
  wires:
  F_res (N.m)/1 -> Add2/2
  Divide/1 -> Mux2/1, Sum/2
  Crankshaft Inertia/1 -> Mux1/1
  Diff_ratio/1 -> Mux1/2
  Mux1/1 -> Equivalent mass/1
  GearLevel_MD/1 -> Mux1/3
  Equivalent mass/1 -> Divide/2
  GL_MD/1 -> GearLevel_MD/1
  V0/1 -> mph-->mps/1
  mph-->mps/1 -> Discrete-Time Integrator/2
  mps-->mph/1 -> Mux/1, Sum1/2, Saturation/1
  F_tractive [N]/1 -> Add2/1
  Discrete-Time Integrator/1 -> mps-->mph/1
  Saturation/1 -> Sum1/1, Mux/2, VESP (MPH)/1
  Add2/1 -> Divide/1
  Sum1/1 -> Scope/2, Gain/1
  Gain/1 -> Sum/1
  Sum/1 -> Mux2/2, Discrete-Time Integrator/1
  Mux/1 -> Scope/1
  Mux2/1 -> Scope/3

== system VehicleModel/Subsystem/Follower vehicle Subsystem/Follow Vehicle/last gear level ==
  In1 : Inport
  Trigger : TriggerPort  VariantControl=Variant
  Out1 : Outport  InitialOutput=1
  wires:
  In1/1 -> Out1/1

== system VehicleModel/Subsystem/Follower vehicle Subsystem/Follow Vehicle/Chunan's Off-delay/OFF Delay ==
  note: IC = ic
  note: IC = -inf
  IN : Inport
  clock : Inport  Port=2
  DELAY : Inport  Port=3
  Enable : EnablePort  PropagateVarSize=During execution
  Chunan's edge detector : Subsystem
  Logical Operator : Logic  Operator=NOT  Inputs=1
  Logical Operator1 : Logic  OutDataTypeStr=boolean
  Logical Operator2 : Logic  Operator=NOT  Inputs=1
  Model : Subsystem  AncestorBlock=spsSampleAndHoldModel/Continuous
  Relational Operator : RelationalOperator  OutDataTypeStr=boolean  RndMeth=Nearest  InputSameDT=on
  Sum : Sum  SaturateOnIntegerOverflow=on  InputSameDT=on  OutDataTypeStr=Inherit: Same as first input
  OUT : Outport
  wires:
  Logical Operator/1 -> Logical Operator1/2
  Relational Operator/1 -> Logical Operator1/1
  Model/1(Out) -> Sum/1
  Sum/1 -> Relational Operator/2
  DELAY/1 -> Sum/2
  Logical Operator1/1 -> Logical Operator2/1
  Logical Operator2/1 -> OUT/1
  IN/1 -> Chunan's edge detector/1(In1), Logical Operator/1
  clock/1 -> Relational Operator/1, Model/1(In)
  Chunan's edge detector/1(Out1) -> Model/2(S)

== system VehicleModel/Subsystem/Follower vehicle Subsystem/Follow Vehicle/Chunan's Off-delay1/OFF Delay ==
  note: IC = ic
  note: IC = -inf
  IN : Inport
  clock : Inport  Port=2
  DELAY : Inport  Port=3
  Enable : EnablePort  PropagateVarSize=During execution
  Chunan's edge detector : Subsystem
  Logical Operator : Logic  Operator=NOT  Inputs=1
  Logical Operator1 : Logic  OutDataTypeStr=boolean
  Logical Operator2 : Logic  Operator=NOT  Inputs=1
  Model : Subsystem  AncestorBlock=spsSampleAndHoldModel/Continuous
  Relational Operator : RelationalOperator  OutDataTypeStr=boolean  RndMeth=Nearest  InputSameDT=on
  Sum : Sum  SaturateOnIntegerOverflow=on  InputSameDT=on  OutDataTypeStr=Inherit: Same as first input
  OUT : Outport
  wires:
  Logical Operator/1 -> Logical Operator1/2
  Relational Operator/1 -> Logical Operator1/1
  Model/1(Out) -> Sum/1
  Sum/1 -> Relational Operator/2
  DELAY/1 -> Sum/2
  Logical Operator1/1 -> Logical Operator2/1
  Logical Operator2/1 -> OUT/1
  IN/1 -> Chunan's edge detector/1(In1), Logical Operator/1
  clock/1 -> Relational Operator/1, Model/1(In)
  Chunan's edge detector/1(Out1) -> Model/2(S)

== system VehicleModel/Subsystem/Follower vehicle Subsystem/Follow Vehicle/DRIVER_RSL/PT1_1 ==
  T_constant : Inport
  in : Inport  Port=2
  T_sample : Inport  Port=3
  map_error_1 : Sum  Inputs=+-  SaturateOnIntegerOverflow=on  InputSameDT=on  OutDataTypeStr=Inherit: Same as first input
  map_error_2 : Sum  Inputs=2  SaturateOnIntegerOverflow=on  InputSameDT=on  OutDataTypeStr=Inherit: Same as first input
  product_1 : Product  Inputs=*/  SaturateOnIntegerOverflow=on  InputSameDT=on  OutDataTypeStr=Inherit: Same as first input
  product_2 : Product  Inputs=**  SaturateOnIntegerOverflow=on  InputSameDT=on  OutDataTypeStr=Inherit: Same as first input
  saturation_1 : Saturate  UpperLimit=1  LowerLimit=0
  unit_delay_1 : UnitDelay  SampleTime=-1
  out : Outport
  wires:
  T_constant/1 -> product_1/2
  T_sample/1 -> product_1/1
  in/1 -> map_error_1/1
  map_error_1/1 -> product_2/2
  product_1/1 -> saturation_1/1
  saturation_1/1 -> product_2/1
  unit_delay_1/1 -> map_error_1/2, map_error_2/2
  map_error_2/1 -> out/1, unit_delay_1/1
  product_2/1 -> map_error_2/1

== system VehicleModel/Subsystem/Follower vehicle Subsystem/Follow Vehicle/DRIVER_RSL/PT1_2 ==
  T_constant : Inport
  in : Inport  Port=2
  T_sample : Inport  Port=3
  map_error_1 : Sum  Inputs=+-  SaturateOnIntegerOverflow=on  InputSameDT=on  OutDataTypeStr=Inherit: Same as first input
  map_error_2 : Sum  Inputs=2  SaturateOnIntegerOverflow=on  InputSameDT=on  OutDataTypeStr=Inherit: Same as first input
  product_1 : Product  Inputs=*/  SaturateOnIntegerOverflow=on  InputSameDT=on  OutDataTypeStr=Inherit: Same as first input
  product_2 : Product  Inputs=**  SaturateOnIntegerOverflow=on  InputSameDT=on  OutDataTypeStr=Inherit: Same as first input
  saturation_1 : Saturate  UpperLimit=1  LowerLimit=0
  unit_delay_1 : UnitDelay  SampleTime=-1
  out : Outport
  wires:
  T_constant/1 -> product_1/2
  T_sample/1 -> product_1/1
  in/1 -> map_error_1/1
  map_error_1/1 -> product_2/2
  product_1/1 -> saturation_1/1
  saturation_1/1 -> product_2/1
  unit_delay_1/1 -> map_error_1/2, map_error_2/2
  map_error_2/1 -> out/1, unit_delay_1/1
  product_2/1 -> map_error_2/1

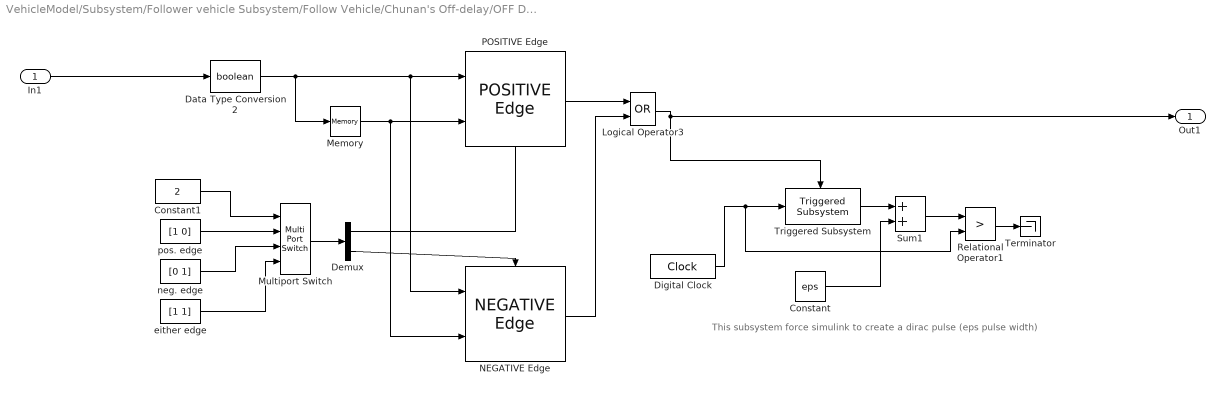
== system VehicleModel/Subsystem/Follower vehicle Subsystem/Follow Vehicle/Chunan's Off-delay/OFF Delay/Chunan's edge detector ==
  note: This subsystem force simulink to create a dirac pulse (eps pulse width)
  In1 : Inport
  Constant : Constant  Value=eps
  Constant1 : Constant  Value=2
  Data Type Conversion2 : DataTypeConversion  OutDataTypeStr=boolean
  Demux : Demux  Outputs=2
  Digital Clock : DigitalClock  SampleTime=-1
  Logical Operator3 : Logic  Operator=OR  OutDataTypeStr=boolean
  Memory : Memory  InheritSampleTime=on  LinearizeAsDelay=on
  Multiport Switch : MultiPortSwitch  SaturateOnIntegerOverflow=on
  NEGATIVE Edge : spsEdgeDetectorModel/Continuous/NEGATIVE Edge
  POSITIVE Edge : spsEdgeDetectorModel/Continuous/POSITIVE Edge
  Relational Operator1 : RelationalOperator  Operator=>  OutDataTypeStr=boolean  RndMeth=Nearest  InputSameDT=on
  Sum1 : Sum  SaturateOnIntegerOverflow=on  InputSameDT=on  OutDataTypeStr=Inherit: Same as first input
  Terminator : Terminator
  Triggered Subsystem : spsEdgeDetectorModel/Continuous/Internal dirac generator/Triggered Subsystem
  either edge : Constant  Value=[1 1]
  neg. edge : Constant  Value=[0 1]
  pos. edge : Constant  Value=[1 0]
  Out1 : Outport
  wires:
  Constant1/1 -> Multiport Switch/1
  Demux/1 -> POSITIVE Edge/Enable
  Demux/2 -> NEGATIVE Edge/Enable
  NEGATIVE Edge/1 -> Logical Operator3/2
  POSITIVE Edge/1 -> Logical Operator3/1
  Data Type Conversion2/1 -> Memory/1, POSITIVE Edge/1, NEGATIVE Edge/1
  either edge/1 -> Multiport Switch/4
  pos. edge/1 -> Multiport Switch/2
  Multiport Switch/1 -> Demux/1
  Memory/1 -> POSITIVE Edge/2, NEGATIVE Edge/2
  In1/1 -> Data Type Conversion2/1
  neg. edge/1 -> Multiport Switch/3
  Logical Operator3/1 -> Out1/1, Triggered Subsystem/Trigger
  Relational Operator1/1 -> Terminator/1
  Digital Clock/1 -> Triggered Subsystem/1, Relational Operator1/2
  Constant/1 -> Sum1/2
  Sum1/1 -> Relational Operator1/1
  Triggered Subsystem/1 -> Sum1/1

== system VehicleModel/Subsystem/Follower vehicle Subsystem/Follow Vehicle/Chunan's Off-delay/OFF Delay/Model ==
  In : Inport
  S : Inport  Port=2
  Data Type Conversion : DataTypeConversion  OutDataTypeStr=boolean
  IC=ic : Memory  InheritSampleTime=on  LinearizeAsDelay=on
  Switch : Switch  Threshold=0.5  SaturateOnIntegerOverflow=on  InputSameDT=on
  Out : Outport  InitialOutput=0
  wires:
  Data Type Conversion/1 -> Switch/2
  Switch/1 -> IC=ic/1, Out/1
  IC=ic/1 -> Switch/3
  In/1 -> Switch/1
  S/1 -> Data Type Conversion/1

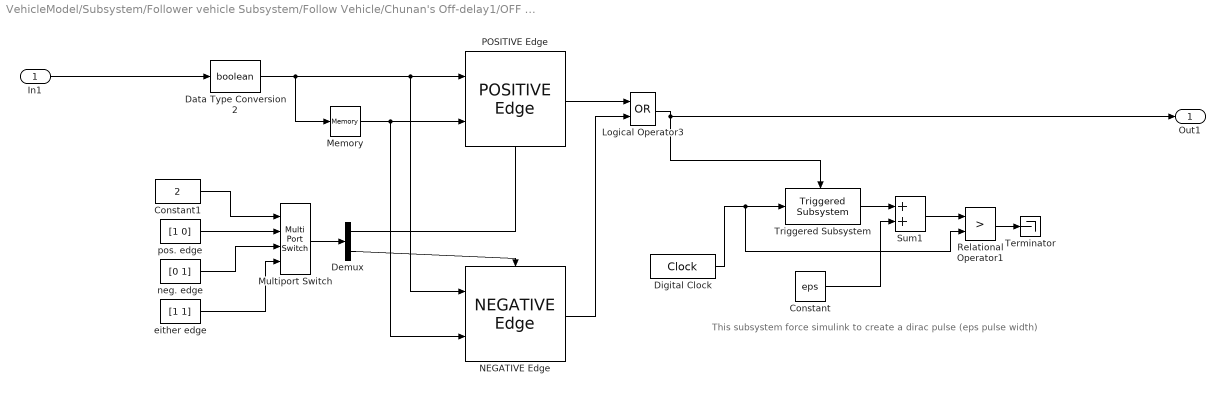
== system VehicleModel/Subsystem/Follower vehicle Subsystem/Follow Vehicle/Chunan's Off-delay1/OFF Delay/Chunan's edge detector ==
  note: This subsystem force simulink to create a dirac pulse (eps pulse width)
  In1 : Inport
  Constant : Constant  Value=eps
  Constant1 : Constant  Value=2
  Data Type Conversion2 : DataTypeConversion  OutDataTypeStr=boolean
  Demux : Demux  Outputs=2
  Digital Clock : DigitalClock  SampleTime=-1
  Logical Operator3 : Logic  Operator=OR  OutDataTypeStr=boolean
  Memory : Memory  InheritSampleTime=on  LinearizeAsDelay=on
  Multiport Switch : MultiPortSwitch  SaturateOnIntegerOverflow=on
  NEGATIVE Edge : spsEdgeDetectorModel/Continuous/NEGATIVE Edge
  POSITIVE Edge : spsEdgeDetectorModel/Continuous/POSITIVE Edge
  Relational Operator1 : RelationalOperator  Operator=>  OutDataTypeStr=boolean  RndMeth=Nearest  InputSameDT=on
  Sum1 : Sum  SaturateOnIntegerOverflow=on  InputSameDT=on  OutDataTypeStr=Inherit: Same as first input
  Terminator : Terminator
  Triggered Subsystem : spsEdgeDetectorModel/Continuous/Internal dirac generator/Triggered Subsystem
  either edge : Constant  Value=[1 1]
  neg. edge : Constant  Value=[0 1]
  pos. edge : Constant  Value=[1 0]
  Out1 : Outport
  wires:
  Constant1/1 -> Multiport Switch/1
  Demux/1 -> POSITIVE Edge/Enable
  Demux/2 -> NEGATIVE Edge/Enable
  NEGATIVE Edge/1 -> Logical Operator3/2
  POSITIVE Edge/1 -> Logical Operator3/1
  Data Type Conversion2/1 -> Memory/1, POSITIVE Edge/1, NEGATIVE Edge/1
  either edge/1 -> Multiport Switch/4
  pos. edge/1 -> Multiport Switch/2
  Multiport Switch/1 -> Demux/1
  Memory/1 -> POSITIVE Edge/2, NEGATIVE Edge/2
  In1/1 -> Data Type Conversion2/1
  neg. edge/1 -> Multiport Switch/3
  Logical Operator3/1 -> Out1/1, Triggered Subsystem/Trigger
  Relational Operator1/1 -> Terminator/1
  Digital Clock/1 -> Triggered Subsystem/1, Relational Operator1/2
  Constant/1 -> Sum1/2
  Sum1/1 -> Relational Operator1/1
  Triggered Subsystem/1 -> Sum1/1

== system VehicleModel/Subsystem/Follower vehicle Subsystem/Follow Vehicle/Chunan's Off-delay1/OFF Delay/Model ==
  In : Inport
  S : Inport  Port=2
  Data Type Conversion : DataTypeConversion  OutDataTypeStr=boolean
  IC=ic : Memory  InheritSampleTime=on  LinearizeAsDelay=on
  Switch : Switch  Threshold=0.5  SaturateOnIntegerOverflow=on  InputSameDT=on
  Out : Outport  InitialOutput=0
  wires:
  Data Type Conversion/1 -> Switch/2
  Switch/1 -> IC=ic/1, Out/1
  IC=ic/1 -> Switch/3
  In/1 -> Switch/1
  S/1 -> Data Type Conversion/1
